simulink model "dof1_paper"  (R2014b)
settings: Solver=ode45  StartTime=0.0  StopTime=50  RelTol=1e-3
undefined symbols (not defined in the file or in its folder): magnitude
libraries: simulink x5
settings Model: Creator=dlr\mish_hr  LastModifiedBy=dlr\mish_hr

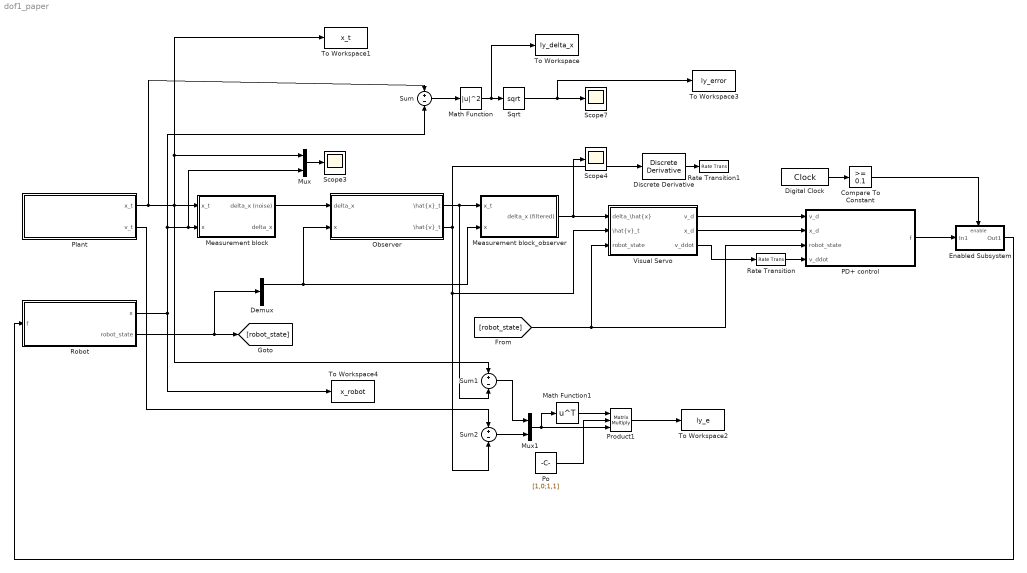
== system dof1_paper ==
  Compare To Constant : simulink/Logic and Bit Operations/Compare To Constant  relop=>=  const=0.1  OutDataTypeStr=boolean
  Demux : Demux  Outputs=2
  Digital Clock : DigitalClock  SampleTime=0.01
  Discrete Derivative : simulink/Discrete/Discrete Derivative  gainval=1.0  ICPrevScaledInput=0.0  InputProcessing=Inherited  OutMin=[]  OutMax=[]  OutDataType=fixdt(1, 16)  OutScaling=2^-10  DoSatur=off
  Enabled Subsystem : Subsystem  TreatAsAtomicUnit=on
  Math Function : Math  Operator=magnitude^2  SaturateOnIntegerOverflow=on
  Math Function1 : Math  Operator=transpose  SaturateOnIntegerOverflow=on
  Measurement block : Subsystem
  Measurement block_observer : Subsystem  TreatAsAtomicUnit=on  SystemSampleTime=0.1
  Mux : Mux  Inputs=2
  Mux1 : Mux  Inputs=2
  Observer : Subsystem  TreatAsAtomicUnit=on  SystemSampleTime=0.1
  PD+ control : Subsystem  TreatAsAtomicUnit=on  SystemSampleTime=0.01
  Plant : Subsystem
  Po : Constant  Value=[1,0;1,1]
  Product1 : Product  Inputs=3  Multiplication=Matrix(*)
  Rate Transition : RateTransition  OutPortSampleTime=.1
  Rate Transition1 : RateTransition  OutPortSampleTime=.1
  Robot : Subsystem
  Scope3 : Scope
      settings: TimeRange=30  SaveName=ScopeData5
  Scope4 : Scope
      settings: TimeRange=30  SaveName=ScopeData12
  Scope7 : Scope
      settings: TimeRange=30  SaveName=ScopeData11
  Sqrt : Sqrt  SaturateOnIntegerOverflow=on
  Sum : Sum  Inputs=+-
  Sum1 : Sum  Inputs=+-
  Sum2 : Sum  Inputs=+-
  To Workspace : ToWorkspace  VariableName=ly_delta_x  SaveFormat=Timeseries  SampleTime=-1
  To Workspace1 : ToWorkspace  VariableName=x_t  SaveFormat=Timeseries  SampleTime=-1
  To Workspace2 : ToWorkspace  VariableName=ly_e  SaveFormat=Timeseries  SampleTime=-1
  To Workspace3 : ToWorkspace  VariableName=ly_error  SaveFormat=Timeseries  SampleTime=-1
  To Workspace4 : ToWorkspace  VariableName=x_robot  SaveFormat=Timeseries  SampleTime=-1
  Visual Servo : Subsystem  TreatAsAtomicUnit=on  SystemSampleTime=0.01
  wires:
  Plant/1(x_t) -> Sum/1, Sum1/1, To Workspace1/1, Mux/1, Measurement block/1(x_t)
  Robot/1(x) -> Sum/2, Mux/2, Measurement block/2(x), To Workspace4/1
  Measurement block/1(delta_x (noise)) -> Observer/1(delta_x)
  Observer/1("\\hat{x}_t") -> Measurement block_observer/1(x_t), Sum1/2
  Measurement block_observer/1(delta_x (filtered)) -> Scope4/1, Visual Servo/1("delta_\\hat{x} ")
  Robot/2(robot_state) -> Demux/1, [robot_state]
  [robot_state] -> Visual Servo/3(robot_state), PD+ control/3(robot_state)
  Demux/1 -> Measurement block_observer/2(x), Observer/2(x)
  Digital Clock/1 -> Compare To Constant/1
  Compare To Constant/1 -> Enabled Subsystem/Enable
  PD+ control/1(f) -> Enabled Subsystem/1(In1)
  Sum/1 -> Math Function/1
  Math Function/1 -> To Workspace/1, Sqrt/1
  Sqrt/1 -> To Workspace3/1, Scope7/1
  Mux/1 -> Scope3/1
  Plant/2("v_t ") -> Sum2/1
  Enabled Subsystem/1(Out1) -> Robot/1(f)
  Visual Servo/3(v_ddot) -> Rate Transition/1
  Sum2/1 -> Mux1/2
  Sum1/1 -> Mux1/1
  Po/1 -> Product1/2
  Math Function1/1 -> Product1/1
  Mux1/1 -> Math Function1/1, Product1/3
  Product1/1 -> To Workspace2/1
  Discrete Derivative/1 -> Rate Transition1/1
  Observer/2("\\hat{v}_t") -> Discrete Derivative/1, Visual Servo/2("\\hat{v}_t"), Sum2/2
  Rate Transition/1 -> PD+ control/4(v_ddot)
  Visual Servo/1(v_d) -> PD+ control/1(v_d)
  Visual Servo/2(x_d) -> PD+ control/2(x_d)

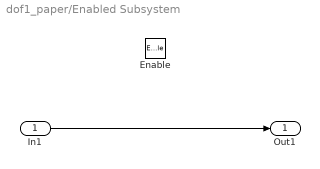
== system dof1_paper/Enabled Subsystem ==
  In1 : Inport
  Enable : EnablePort
  Out1 : Outport
  wires:
  In1/1 -> Out1/1

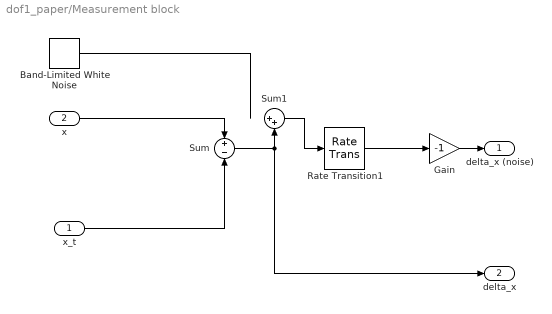
== system dof1_paper/Measurement block ==
  x_t : Inport
  x : Inport  Port=2
  Band-Limited White Noise : simulink/Sources/Band-Limited White Noise  Cov=1e-4  Ts=0.1  seed=[23341]
  Gain : Gain  Gain=-1
  Rate Transition1 : RateTransition  OutPortSampleTime=0.1
  Sum : Sum  Inputs=+-
  Sum1 : Sum  Inputs=|++
  delta_x (noise) : Outport
  "delta_x " : Outport  Port=2
  wires:
  x_t/1 -> Sum/2
  Sum1/1 -> Rate Transition1/1
  Band-Limited White Noise/1 -> ?
  x/1 -> Sum/1
  Rate Transition1/1 -> Gain/1
  Gain/1 -> delta_x (noise)/1
  Sum/1 -> Sum1/2, "delta_x "/1

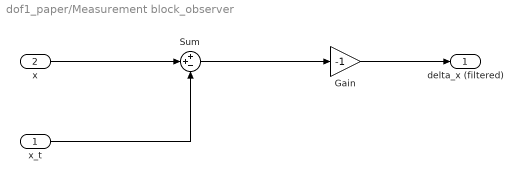
== system dof1_paper/Measurement block_observer ==
  x_t : Inport
  x : Inport  Port=2
  Gain : Gain  Gain=-1
  Sum : Sum  Inputs=++-
  delta_x (filtered) : Outport
  wires:
  Gain/1 -> delta_x (filtered)/1
  Sum/1 -> Gain/1
  x/1 -> Sum/2
  x_t/1 -> Sum/3

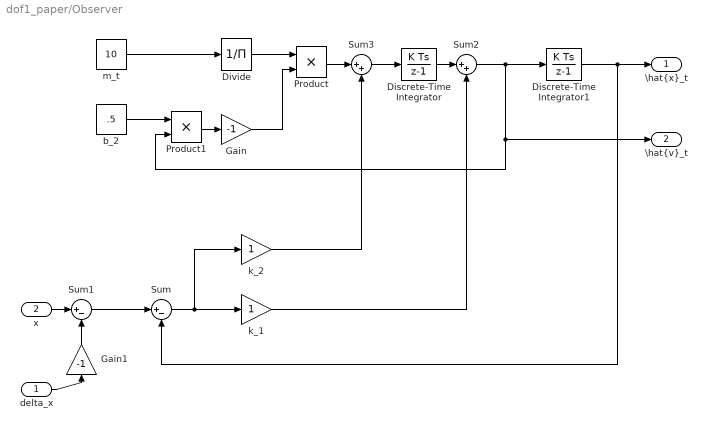
== system dof1_paper/Observer ==
  delta_x : Inport
  x : Inport  Port=2
  Discrete-Time Integrator : DiscreteIntegrator  InitialConditionSetting=State (most efficient)  SampleTime=-1
  Discrete-Time Integrator1 : DiscreteIntegrator  InitialConditionSetting=State (most efficient)  SampleTime=-1
  Divide : Product  Inputs=/
  Gain : Gain  Gain=-1
  Gain1 : Gain  Gain=-1
  Product : Product
  Product1 : Product
  Sum : Sum  Inputs=|+-
  Sum1 : Sum  Inputs=|+-
  Sum2 : Sum  Inputs=|++
  Sum3 : Sum  Inputs=|++
  b_2 : Constant  Value=.5
  k_1 : Gain
  k_2 : Gain
  m_t : Constant  Value=10
  "\\hat{x}_t" : Outport
  "\\hat{v}_t" : Outport  Port=2
  wires:
  Product1/1 -> Gain/1
  Discrete-Time Integrator1/1 -> Sum/2, "\\hat{x}_t"/1
  Sum3/1 -> Discrete-Time Integrator/1
  Divide/1 -> Product/1
  Sum2/1 -> Discrete-Time Integrator1/1, Product1/2, "\\hat{v}_t"/1
  m_t/1 -> Divide/1
  b_2/1 -> Product1/1
  Gain/1 -> Product/2
  Sum1/1 -> Sum/1
  Sum/1 -> k_2/1, k_1/1
  Discrete-Time Integrator/1 -> Sum2/1
  k_1/1 -> Sum2/2
  k_2/1 -> Sum3/2
  Product/1 -> Sum3/1
  x/1 -> Sum1/1
  delta_x/1 -> Gain1/1
  Gain1/1 -> Sum1/2

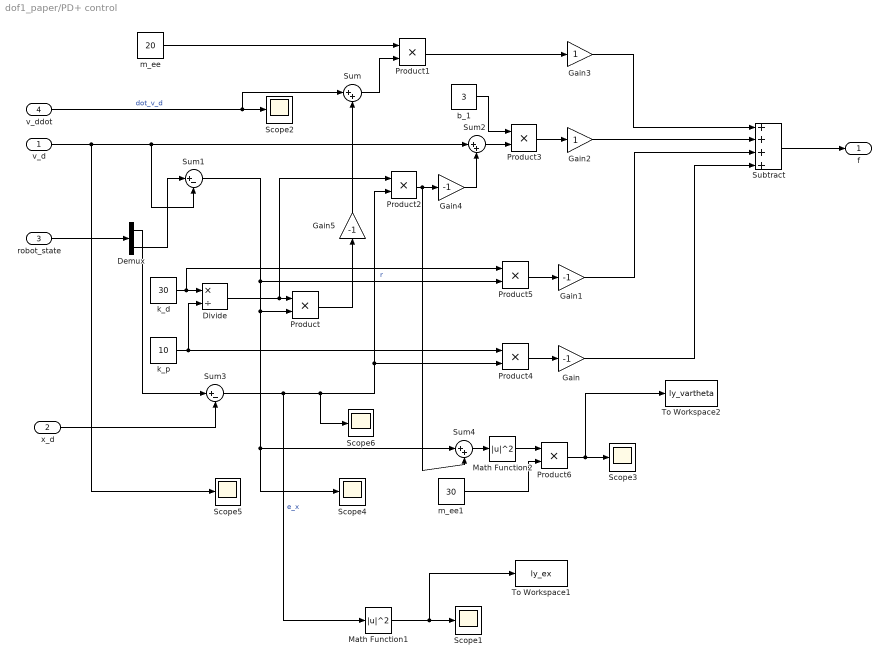
== system dof1_paper/PD+ control ==
  v_d : Inport
  x_d : Inport  Port=2
  robot_state : Inport  Port=3
  v_ddot : Inport  Port=4
  Demux : Demux  Outputs=2
  Divide : Product  Inputs=*/
  Gain{,1,4..5} (4 alike) : Gain  Gain=-1
  Gain2 : Gain
  Gain3 : Gain
  Math Function1 : Math  Operator=magnitude^2  SaturateOnIntegerOverflow=on
  Math Function2 : Math  Operator=magnitude^2  SaturateOnIntegerOverflow=on
  Product{,1..6} (7 alike) : Product
  Scope{1..6} (6 alike) : Scope
      Scope1 settings: TimeRange=30  SaveName=ScopeData2
      Scope2 settings: TimeRange=30  SaveName=ScopeData3
      Scope3 settings: TimeRange=30  SaveName=ScopeData4
      Scope4 settings: TimeRange=49.99  YMin=-0.5358447488584475  YMax=0.1970319634703197  SaveName=ScopeData6
      Scope5 settings: TimeRange=49.99  YMin=-0.5358447488584475  YMax=0.1970319634703197  SaveName=ScopeData10
      Scope6 settings: TimeRange=49.99  YMin=-0.5358447488584475  YMax=0.1970319634703197  SaveName=ScopeData13
  Subtract : Sum  Inputs=++++
  Sum : Sum  Inputs=|++
  Sum1 : Sum  Inputs=|+-
  Sum2 : Sum  Inputs=|++
  Sum3 : Sum  Inputs=|+-
  Sum4 : Sum  Inputs=|++
  To Workspace1 : ToWorkspace  VariableName=ly_ex  SaveFormat=Timeseries  SampleTime=-1
  To Workspace2 : ToWorkspace  VariableName=ly_vartheta  SaveFormat=Timeseries  SampleTime=-1
  b_1 : Constant  Value=3
  k_d : Constant  Value=30
  k_p : Constant  Value=10
  m_ee : Constant  Value=20
  m_ee1 : Constant  Value=30
  f : Outport
  wires:
  v_d/1 -> Scope5/1, Sum1/2, Sum2/1
  k_d/1 -> Product5/1, Divide/1
  k_p/1 -> Product4/1, Divide/2
  v_ddot/1 -> Sum/1, Scope2/1  "dot_v_d"
  Divide/1 -> Product2/1, Product/1
  robot_state/1 -> Demux/1
  Demux/2 -> Sum1/1
  Sum1/1 -> Product5/2, Scope4/1, Sum4/1, Product/2  "r"
  Product/1 -> Gain5/1
  Sum/1 -> Product1/2
  m_ee/1 -> Product1/1
  Demux/1 -> Sum3/1
  x_d/1 -> Sum3/2
  Sum3/1 -> Math Function1/1, Scope6/1, Product4/2, Product2/2  "e_x"
  Product2/1 -> Gain4/1, Sum4/2
  Sum2/1 -> Product3/2
  b_1/1 -> Product3/1
  Product4/1 -> Gain/1
  Product5/1 -> Gain1/1
  Product1/1 -> Gain3/1
  Product3/1 -> Gain2/1
  Gain1/1 -> Subtract/3
  Gain/1 -> Subtract/4
  Subtract/1 -> f/1
  Gain2/1 -> Subtract/2
  Gain3/1 -> Subtract/1
  Math Function1/1 -> To Workspace1/1, Scope1/1
  Sum4/1 -> Math Function2/1
  m_ee1/1 -> Product6/2
  Math Function2/1 -> Product6/1
  Product6/1 -> To Workspace2/1, Scope3/1
  Gain4/1 -> Sum2/2
  Gain5/1 -> Sum/2

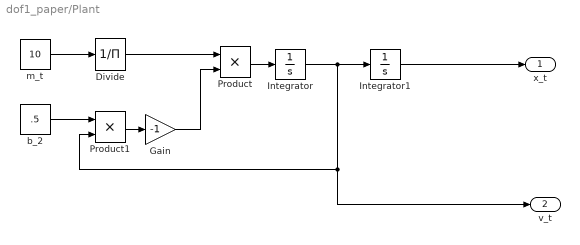
== system dof1_paper/Plant ==
  Divide : Product  Inputs=/
  Gain : Gain  Gain=-1
  Integrator : Integrator  InitialCondition=.4
  Integrator1 : Integrator  InitialCondition=5
  Product : Product
  Product1 : Product
  b_2 : Constant  Value=.5
  m_t : Constant  Value=10
  x_t : Outport
  "v_t " : Outport  Port=2
  wires:
  Product1/1 -> Gain/1
  Integrator1/1 -> x_t/1
  Product/1 -> Integrator/1
  Divide/1 -> Product/1
  m_t/1 -> Divide/1
  b_2/1 -> Product1/1
  Gain/1 -> Product/2
  Integrator/1 -> Integrator1/1, "v_t "/1, Product1/2

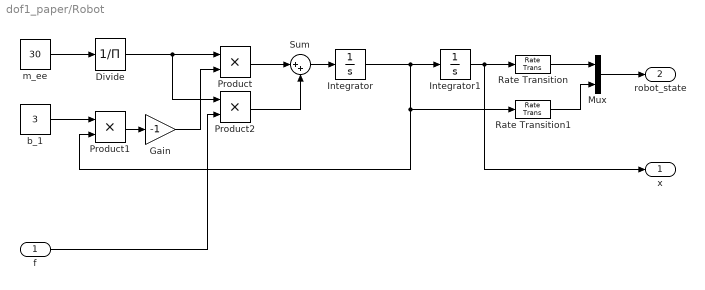
== system dof1_paper/Robot ==
  f : Inport
  Divide : Product  Inputs=/
  Gain : Gain  Gain=-1
  Integrator : Integrator
  Integrator1 : Integrator
  Mux : Mux  Inputs=2
  Product : Product
  Product1 : Product
  Product2 : Product
  Rate Transition : RateTransition  OutPortSampleTime=0.01
  Rate Transition1 : RateTransition  OutPortSampleTime=0.01
  Sum : Sum  Inputs=|++
  b_1 : Constant  Value=3
  m_ee : Constant  Value=30
  x : Outport
  robot_state : Outport  Port=2
  wires:
  Gain/1 -> Product/2
  b_1/1 -> Product1/1
  m_ee/1 -> Divide/1
  Divide/1 -> Product2/1, Product/1
  Sum/1 -> Integrator/1
  Integrator1/1 -> x/1, Rate Transition/1
  Product1/1 -> Gain/1
  Product/1 -> Sum/1
  f/1 -> Product2/2
  Product2/1 -> Sum/2
  Rate Transition/1 -> Mux/1
  Rate Transition1/1 -> Mux/2
  Integrator/1 -> Rate Transition1/1, Product1/2, Integrator1/1
  Mux/1 -> robot_state/1

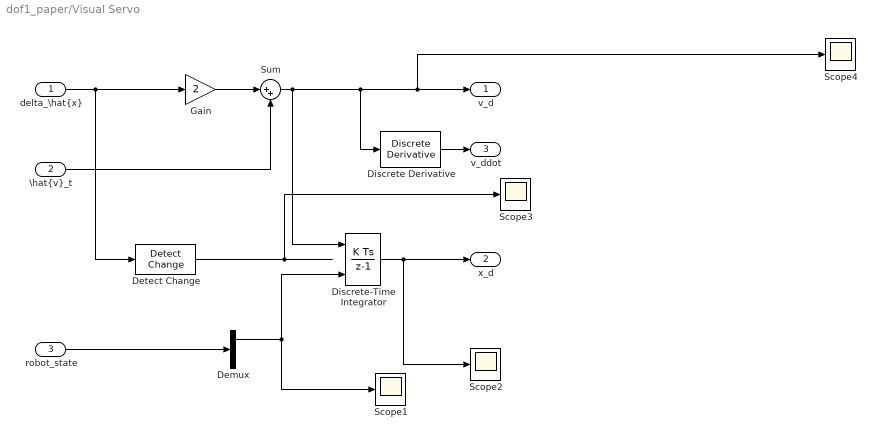
== system dof1_paper/Visual Servo ==
  "delta_\\hat{x} " : Inport
  "\\hat{v}_t" : Inport  Port=2
  robot_state : Inport  Port=3
  Demux : Demux  Outputs=2
  Detect Change : simulink/Logic and Bit Operations/Detect Change  vinit=0  InputProcessing=Inherited  OutDataTypeStr=boolean
  Discrete Derivative : simulink/Discrete/Discrete Derivative  gainval=1.0  ICPrevScaledInput=0.0  InputProcessing=Inherited  OutMin=[]  OutMax=[]  OutDataType=fixdt(1, 16)  OutScaling=2^-10  DoSatur=off
  Discrete-Time Integrator : DiscreteIntegrator  ExternalReset=rising  InitialConditionSource=external  InitialConditionSetting=State (most efficient)  SampleTime=-1
  Gain : Gain  Gain=2
  Scope{1..4} (4 alike) : Scope
      Scope1 settings: TimeRange=30  SaveName=ScopeData8
      Scope2 settings: TimeRange=30  SaveName=ScopeData7
      Scope3 settings: TimeRange=30  SaveName=ScopeData9
      Scope4 settings: TimeRange=30
  Sum : Sum  Inputs=|++
  v_d : Outport
  x_d : Outport  Port=2
  v_ddot : Outport  Port=3
  wires:
  Sum/1 -> Scope4/1, v_d/1, Discrete Derivative/1, Discrete-Time Integrator/1
  "delta_\\hat{x} "/1 -> Detect Change/1, Gain/1
  Gain/1 -> Sum/1
  "\\hat{v}_t"/1 -> Sum/2
  Discrete-Time Integrator/1 -> Scope2/1, x_d/1
  Detect Change/1 -> Scope3/1
  robot_state/1 -> Demux/1
  Demux/1 -> Scope1/1, Discrete-Time Integrator/3
  Discrete Derivative/1 -> v_ddot/1
